simulink model "BLDCMODELTOTALNEURON"  (R2020a)
settings: Solver=ode45  StartTime=0.0  StopTime=2  RelTol=1e-3  EnableMultiTasking=on
InitFcn:
  | clc;
StopFcn:
  | clc;
undefined symbols (not defined in the file): sigbuilder_block, Ts
libraries: neural x55, fl_lib x14, nesl_utility x14, simulink x7, spsIGBTDiodeLib x6, spsVoltageMeasurementLib x3, powerlib_extras x1, spsControlledVoltageSourceLib x1, spsGroundLib x1, spsThreePhaseVIMeasurementLib x1, spspowerguiLib x1
(part 1 of 3)
Description:
  | This simulink model simulates the speed control of permanent magnet
  | brush less DC motor. Complete dynamic model of brush-less DC motor
  | was developed and simulated. Conventional PI controller was employed
  | for speed loop.
  | 
  | Syed Abdul Rahman Kashif
  | EED, UET, Lahore
settings Model: Creator=AbdulRahman  LastModifiedBy=HP
settings SolverCC: ZeroCrossAlgorithm=Adaptive
settings DataIOCC: LimitDataPoints=on  SaveFormat=Array  ReturnWorkspaceOutputs=off
settings OptimizationCC: ExpressionDepthLimit=2147483647  LifeSpan=inf
settings DebuggingCC: UnderspecifiedInitializationDetection=Classic  MergeDetectMultiDrivingBlocksExec=none  SolverPrmCheckMsg=warning  StateNameClashWarn=warning  SFUnexpectedBacktrackingDiag=warning  SFNoUnconditionalDefaultTransitionDiag=warning  ArithmeticOperatorsInVariantConditions=warning
settings HardwareCC: ProdBitPerPointer=32  ProdBitPerSizeT=32  ProdBitPerPtrDiffT=32  ProdLargestAtomicFloat=None  ProdIntDivRoundTo=Undefined  ProdEndianess=Unspecified  ProdWordSize=32  ProdHWDeviceType=32-bit Generic
settings ModelReferenceCC: PropagateSignalLabelsOutOfModel=off
settings SFSimCC: SimUseLocalCustomCode=off  CustomCodeUndefinedFunction=UseInterfaceOnly
settings RTWCC: RTWUseLocalCustomCode=off
settings CodeAppCC: StateflowObjectComments=on
settings GRTTargetCC: TargetLangStandard=C89/C90 (ANSI)
settings ConfigComp: CovMetricSettings=dw  CovSaveCumulativeToWorkspaceVar=on  CovSaveSingleToWorkspaceVar=on  CovExternalEMLEnable=off
settings SimscapeCC: SimscapeNormalizeSystem=off

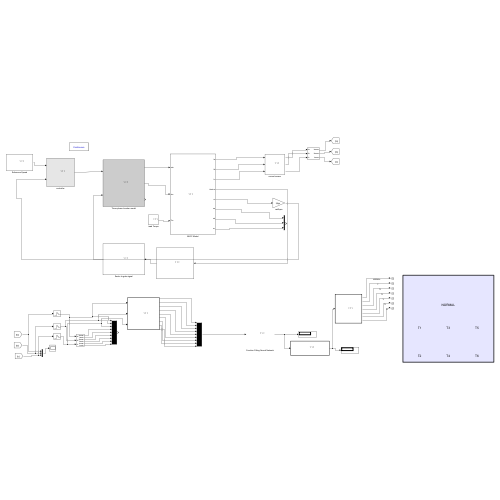
[thumbnail: Simulink's stored preview of the top-level diagram]
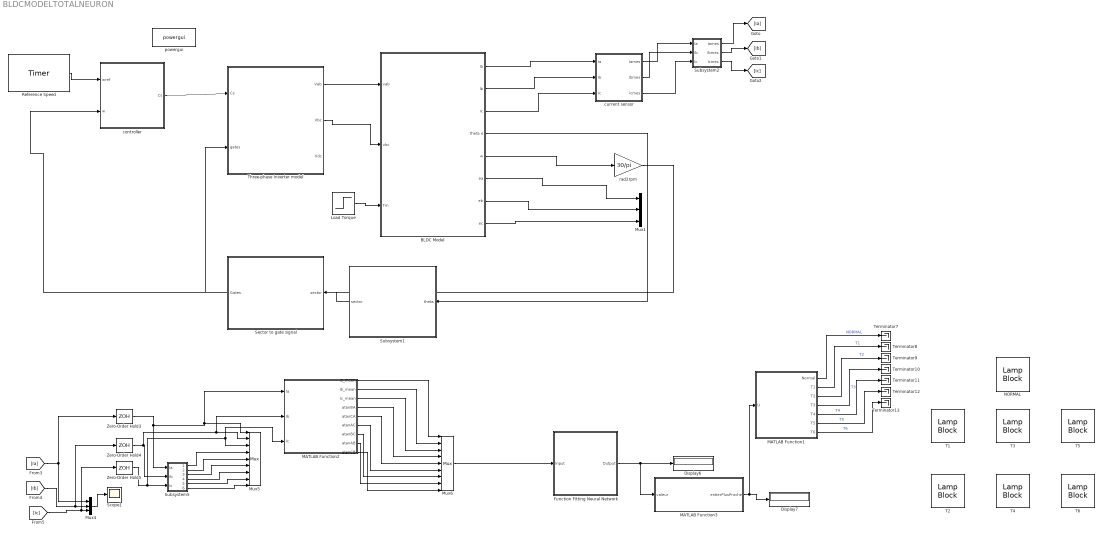
== system BLDCMODELTOTALNEURON ==
  BLDC Model : Subsystem
      mask Display: image(imread('C:\Users\HP\Desktop\2EEIN\PFATOTALYEAR\brush.png'))
  Display6 : Display
  Display7 : Display
  Function Fitting Neural Network : Subsystem
      mask help: Function Fitting Neural Network
      mask Display: image(imread('C:\Users\HP\Desktop\pythonpfa\neuron.png'))
  Load Torque : Step  Time=0.2  After=2  SampleTime=0
      mask Display: image(imread('C:\Users\HP\Desktop\2EEIN\PFATOTALYEAR\tor.png'))
  MATLAB Function1 : MATLAB Function  TreatAsAtomicUnit=on
  MATLAB Function2 : MATLAB Function  TreatAsAtomicUnit=on
  MATLAB Function3 : MATLAB Function  TreatAsAtomicUnit=on
  Mux1 : Mux  Inputs=3
  Mux4 : Mux  Inputs=3
  Mux5 : Mux  Inputs=9
  Mux6 : Mux  Inputs=9
  NORMAL : LampBlock
  Reference Speed : powerlib_extras/Control  Blocks/Timer  t=[0]  e=[1500]  mask(Timer){}
      settings: SourceProductBaseCode=PS
      mask Display:
      | % This is a new mask on top of the base mask.
      | % Use "View base mask" link below to see the base mask.
      | image(imread('C:\Users\HP\Desktop\2EEIN\PFATOTALYEAR\acc.png'))
  Scope1 : Scope
  Sector to gate signal : Subsystem
      mask Display: image(imread('C:\Users\HP\Desktop\2EEIN\PFATOTALYEAR\decoder.png'))
  Subsystem1 : Subsystem
      mask Display: image(imread('C:\Users\HP\Desktop\2EEIN\PFATOTALYEAR\sensor.png'))
  Subsystem2 : Subsystem
  Subsystem5 : Subsystem
  T{1..6} (6 alike) : LampBlock
  Terminator{7..13} (7 alike) : Terminator
  Three-phase Inverter model : Subsystem
      mask Display: image(imread('C:\Users\HP\Desktop\2EEIN\PFATOTALYEAR\threephase.png'))
  Zero-Order Hold3 : ZeroOrderHold  SampleTime=-1
  Zero-Order Hold4 : ZeroOrderHold  SampleTime=-1
  Zero-Order Hold5 : ZeroOrderHold  SampleTime=-1
  controller : Subsystem
      mask Display: image(imread('C:\Users\HP\Desktop\2EEIN\PFATOTALYEAR\pidcont.png'))
  current sensor : Subsystem
      mask Display: image(imread('C:\Users\HP\Desktop\2EEIN\PFATOTALYEAR\current.png'))
  powergui : spspowerguiLib/powergui  Priority=2  SimulationMode=Continuous  SampleTime=Ts  frequency=60  Iterations=50  frequencyindice=0  Pbase=100e6  ErrMax=1e-4  UnitsV=kV  UnitsW=MW  buscounter=0  FunctionMessages=off  echomessages=off  EnableUseOfTLC=off  CurrentSourceSwitches=off  DisableSnubberDevices=off  DisableRonSwitches=off  DisableVfSwitches=off  DisplayEquations=off  AutomaticDiscreteSolvers=off  SolverType=Tustin  Interpol=off  ExternalGateDelay=off  methode=off  Ts=0  x0status=blocks  SPID=off  SwTol=0  HookPort=off  NonlinearTolerance=1e-4  nMaxIteration=100  ContinueOnMaxIteration=off  RestoreLinks=warning  ResistiveCurrentMeasurement=off  Frange=[0:2:500]  Ylog=off  Xlog=on  ShowGrid=off  save=off  variable=ZData  structure=0  ZoomFFT=on  StartTime=0.0  cycles=1  DisplayStyle=1  fundamental=60  FreqAxis=off  MaxFrequency=1000  frequencyindicesteady=1  RmsSteady=1  display=off
  rad2rpm : Gain  Gain=30/pi
  wires:
  Subsystem1/1(sector) -> Sector to gate signal/1(sector)
  rad2rpm/1 -> controller/2(w)
  Reference Speed/1 -> controller/1(wref)
  Load Torque/1 -> BLDC Model/3(Tm)
  BLDC Model/5(w) -> rad2rpm/1
  BLDC Model/4(theta e) -> Subsystem1/1(theta)
  BLDC Model/6(ea) -> Mux1/1
  BLDC Model/7(eb) -> Mux1/2
  BLDC Model/8(ec) -> Mux1/3
  Sector to gate signal/1(Gates) -> Three-phase Inverter model/2(gates)
  controller/1(Cs) -> Three-phase Inverter model/1(Cs)
  Three-phase Inverter model/2(Vbc) -> BLDC Model/2(vbc)
  Three-phase Inverter model/1(Vab) -> BLDC Model/1(vab)
  BLDC Model/1(Ia) -> current sensor/1(Ia)
  BLDC Model/2(Ib) -> current sensor/2(Ib)
  BLDC Model/3(Ic) -> current sensor/3(Ic)
  current sensor/2(Ibmes) -> Subsystem2/2(Ib)
  Subsystem2/3(Icmes) -> [Ic]
  Subsystem2/1(Iames) -> [Ia]
  Subsystem2/2(Ibmes) -> [Ib]
  current sensor/1(Iames) -> Subsystem2/1(Ia)
  current sensor/3(Icmes) -> Subsystem2/3(Ic)
  Function Fitting Neural Network/1(Output) -> MATLAB Function3/1(valeur), Display6/1
  MATLAB Function2/2(Ib_mean) -> Mux6/2
  Zero-Order Hold3/1 -> MATLAB Function2/1(Ia), Mux5/1, Subsystem5/1(Ia)
  Zero-Order Hold4/1 -> MATLAB Function2/2(Ib), Mux5/2, Subsystem5/2(Ib)
  MATLAB Function2/3(Ic_mean) -> Mux6/3
  Subsystem5/3(Ibmax) -> Mux5/6
  Subsystem5/6(Icmin) -> Mux5/9
  [Ia] -> Zero-Order Hold3/1, Mux4/1
  [Ib] -> Zero-Order Hold4/1, Mux4/2
  Mux4/1 -> Scope1/1
  Mux6/1 -> Function Fitting Neural Network/1(Input)
  MATLAB Function2/6(atanAC) -> Mux6/6
  MATLAB Function2/5(atanCA) -> Mux6/5
  MATLAB Function2/4(atanBA) -> Mux6/4
  Zero-Order Hold5/1 -> MATLAB Function2/3(Ic), Mux5/3, Subsystem5/3(Ic)
  MATLAB Function2/9(atanCB) -> Mux6/9
  [Ic] -> Zero-Order Hold5/1, Mux4/3
  Subsystem5/4(Ibmin) -> Mux5/7
  Subsystem5/5(icmax) -> Mux5/8
  Subsystem5/1(Iamax) -> Mux5/4
  MATLAB Function2/7(atanBC) -> Mux6/7
  MATLAB Function2/8(atanAB) -> Mux6/8
  Subsystem5/2(Iamin) -> Mux5/5
  MATLAB Function2/1(Ia_mean) -> Mux6/1
  MATLAB Function3/1(entierPlusProche) -> MATLAB Function1/1(U), Display7/1
  MATLAB Function1/6(T5) -> Terminator12/1  "T5"
  MATLAB Function1/4(T3) -> Terminator10/1  "T3"
  MATLAB Function1/2(T1) -> Terminator8/1  "T1"
  MATLAB Function1/3(T2) -> Terminator9/1  "T2"
  MATLAB Function1/1(Normal) -> Terminator7/1  "NORMAL"
  MATLAB Function1/7(T6) -> Terminator13/1  "T6"
  MATLAB Function1/5(T4) -> Terminator11/1  "T4"

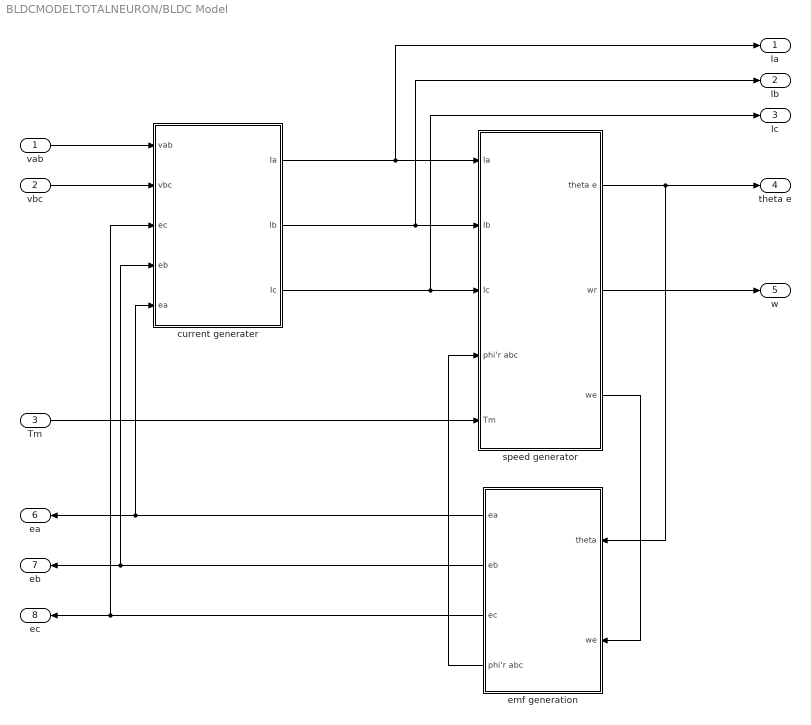
== system BLDCMODELTOTALNEURON/BLDC Model ==
  vab : Inport
  vbc : Inport  Port=2
  Tm : Inport  Port=3
  current generater : Subsystem
  emf generation : Subsystem
  speed generator : Subsystem
  Ia : Outport
  Ib : Outport  Port=2
  Ic : Outport  Port=3
  theta e : Outport  Port=4
  w : Outport  Port=5
  ea : Outport  Port=6
  eb : Outport  Port=7
  ec : Outport  Port=8
  wires:
  vbc/1 -> current generater/2(vbc)
  current generater/1(Ia) -> Ia/1, speed generator/1(Ia)
  current generater/2(Ib) -> Ib/1, speed generator/2(Ib)
  current generater/3(Ic) -> speed generator/3(Ic), Ic/1
  speed generator/1(theta e) -> emf generation/1(theta), theta e/1
  Tm/1 -> speed generator/5(Tm)
  speed generator/2(wr) -> w/1
  emf generation/1(ea) -> ea/1, current generater/5(ea)
  emf generation/2(eb) -> eb/1, current generater/4(eb)
  emf generation/3(ec) -> ec/1, current generater/3(ec)
  emf generation/4(phi'r abc) -> speed generator/4(phi'r abc)
  speed generator/3(we) -> emf generation/2(we)
  vab/1 -> current generater/1(vab)

== system BLDCMODELTOTALNEURON/Function Fitting Neural Network ==
  Input : Inport  PortDimensions=9
      mask Display: e = 0.06;c1 = [120 230 180]/255;c2 = ([120 230 180]+0)/(256+128);c3 = ([120 230 180]+128)/(256+128);patch([0 1 1 0],[0 0 1 1],c1);patch([0 1 1 1-e 1-e 0+e],[0 0 1 1-e 0+e 0+e],c2);patch([0 0 1 1-e 0+e 0+e],[0 1 1 1-e 1-e 0+e],c3);plot([0 1 1 0 0],[0 0 1 1 0]);
  Layer 1 : Subsystem
      mask Display: e = 0.06;c1 = [120 150 230]/255;c2 = ([120 150 230]+0)/383;c3 = ([120 150 230]+128)/383;patch([0 1 1 0],[0 0 1 1],c1);patch([0 1 1 1-e 1-e 0+e],[0 0 1 1-e 0+e 0+e],c2);patch([0 0 1 1-e 0+e 0+e],[0 1 1 1-e 1-e 0+e],c3);plot([0 1 1 0 0],[0 0 1 1 0]);
  Layer 2 : Subsystem
      mask Display: e = 0.06;c1 = [120 150 230]/255;c2 = ([120 150 230]+0)/383;c3 = ([120 150 230]+128)/383;patch([0 1 1 0],[0 0 1 1],c1);patch([0 1 1 1-e 1-e 0+e],[0 0 1 1-e 0+e 0+e],c2);patch([0 0 1 1-e 0+e 0+e],[0 1 1 1-e 1-e 0+e],c3);plot([0 1 1 0 0],[0 0 1 1 0]);
  Process Input 1 : Subsystem
      mask Display: e = 0.06;c1 = [120 150 230]/255;c2 = ([120 150 230]+0)/383;c3 = ([120 150 230]+128)/383;patch([0 1 1 0],[0 0 1 1],c1);patch([0 1 1 1-e 1-e 0+e],[0 0 1 1-e 0+e 0+e],c2);patch([0 0 1 1-e 0+e 0+e],[0 1 1 1-e 1-e 0+e],c3);plot([0 1 1 0 0],[0 0 1 1 0]);
  Process Output 1 : Subsystem
      mask Display: e = 0.06;c1 = [120 150 230]/255;c2 = ([120 150 230]+0)/383;c3 = ([120 150 230]+128)/383;patch([0 1 1 0],[0 0 1 1],c1);patch([0 1 1 1-e 1-e 0+e],[0 0 1 1-e 0+e 0+e],c2);patch([0 0 1 1-e 0+e 0+e],[0 1 1 1-e 1-e 0+e],c3);plot([0 1 1 0 0],[0 0 1 1 0]);
  Output : Outport  InitialOutput=0
      mask Display: e = 0.06;c1 = [120 230 180]/255;c2 = ([120 230 180]+0)/(256+128);c3 = ([120 230 180]+128)/(256+128);patch([0 1 1 0],[0 0 1 1],c1);patch([0 1 1 1-e 1-e 0+e],[0 0 1 1-e 0+e 0+e],c2);patch([0 0 1 1-e 0+e 0+e],[0 1 1 1-e 1-e 0+e],c3);plot([0 1 1 0 0],[0 0 1 1 0]);
  wires:
  Input/1 -> Process Input 1/1(x)
  Process Output 1/1(y) -> Output/1
  Process Input 1/1(p) -> Layer 1/1("p{1}")
  Layer 1/1("a{1}") -> [feedback1]
  [feedback1] -> Layer 2/1("a{1} ")
  Layer 2/1("a{2}") -> Process Output 1/1(a)

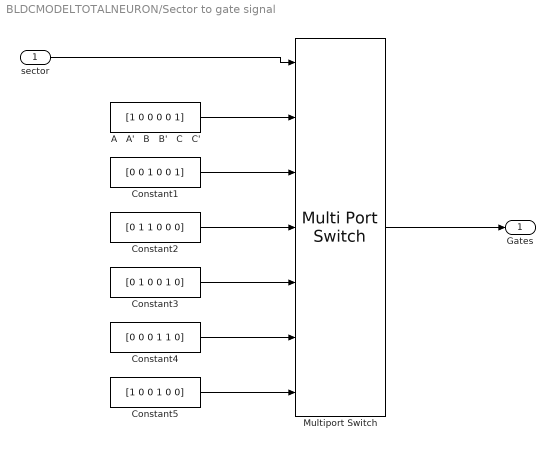
== system BLDCMODELTOTALNEURON/Sector to gate signal ==
  sector : Inport
  A   A'   B   B'   C   C' : Constant  Value=[1 0 0 0 0 1]  VectorParams1D=off
  Constant1 : Constant  Value=[0 0 1 0 0 1]  VectorParams1D=off
  Constant2 : Constant  Value=[0 1 1 0 0 0]  VectorParams1D=off
  Constant3 : Constant  Value=[0 1 0 0 1 0]  VectorParams1D=off
  Constant4 : Constant  Value=[0 0 0 1 1 0]  VectorParams1D=off
  Constant5 : Constant  Value=[1 0 0 1 0 0]  VectorParams1D=off
  Multiport Switch : MultiPortSwitch  Inputs=6
  Gates : Outport
  wires:
  Multiport Switch/1 -> Gates/1
  A   A'   B   B'   C   C'/1 -> Multiport Switch/2
  Constant1/1 -> Multiport Switch/3
  Constant2/1 -> Multiport Switch/4
  Constant3/1 -> Multiport Switch/5
  Constant4/1 -> Multiport Switch/6
  Constant5/1 -> Multiport Switch/7
  sector/1 -> Multiport Switch/1

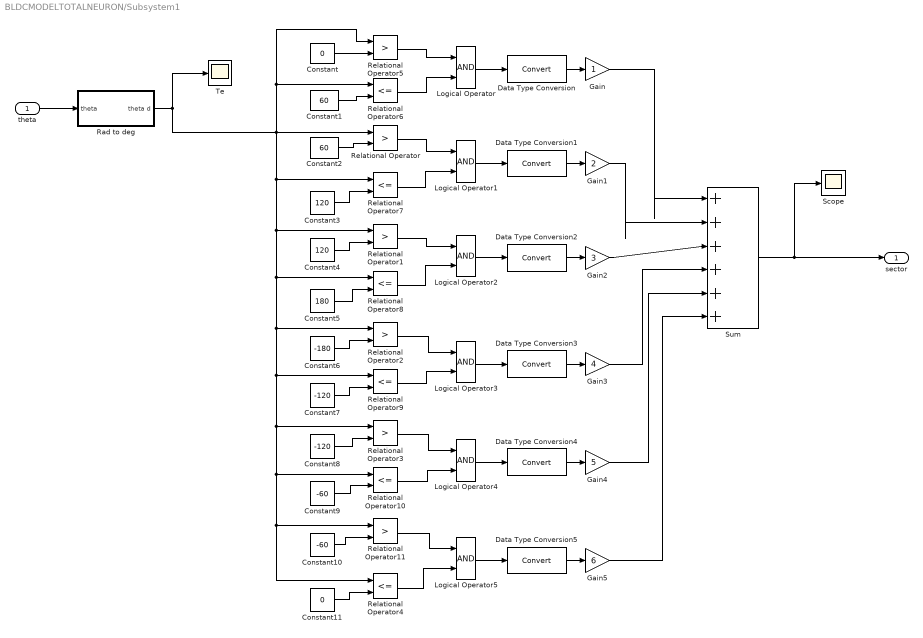
== system BLDCMODELTOTALNEURON/Subsystem1 ==
  theta : Inport
  Constant : Constant  Value=0
  Constant1 : Constant  Value=60
  Constant10 : Constant  Value=-60
  Constant11 : Constant  Value=0
  Constant2 : Constant  Value=60
  Constant3 : Constant  Value=120
  Constant4 : Constant  Value=120
  Constant5 : Constant  Value=180
  Constant6 : Constant  Value=-180
  Constant7 : Constant  Value=-120
  Constant8 : Constant  Value=-120
  Constant9 : Constant  Value=-60
  Data Type Conversion{,1..5} (6 alike) : DataTypeConversion
  Gain : Gain
  Gain1 : Gain  Gain=2
  Gain2 : Gain  Gain=3
  Gain3 : Gain  Gain=4
  Gain4 : Gain  Gain=5
  Gain5 : Gain  Gain=6
  Logical Operator{,1..5} (6 alike) : Logic  AllPortsSameDT=off  OutDataTypeStr=boolean
  Rad to deg : Subsystem
  Relational Operator{,1..3,5,11} (6 alike) : RelationalOperator  Operator=>  OutDataTypeStr=boolean  ZeroCross=off  RndMeth=Nearest
  Relational Operator{4,6..10} (6 alike) : RelationalOperator  Operator=<=  OutDataTypeStr=boolean  ZeroCross=off  RndMeth=Nearest
  Scope : Scope
  Sum : Sum  Inputs=|++++++
  Te : Scope
  sector : Outport
  wires:
  Sum/1 -> sector/1, Scope/1
  theta/1 -> Rad to deg/1(theta)
  Constant/1 -> Relational Operator5/2
  Constant1/1 -> Relational Operator6/2
  Constant2/1 -> Relational Operator/2
  Constant3/1 -> Relational Operator7/2
  Rad to deg/1(theta d) -> Relational Operator5/1, Relational Operator6/1, Relational Operator4/1, Relational Operator11/1, Relational Operator10/1, Relational Operator3/1, Relational Operator9/1, Relational Operator2/1, Relational Operator8/1, Relational Operator1/1, Relational Operator7/1, Relational Operator/1, Te/1
  Constant5/1 -> Relational Operator8/2
  Constant6/1 -> Relational Operator2/2
  Constant7/1 -> Relational Operator9/2
  Constant8/1 -> Relational Operator3/2
  Constant9/1 -> Relational Operator10/2
  Constant10/1 -> Relational Operator11/2
  Constant11/1 -> Relational Operator4/2
  Constant4/1 -> Relational Operator1/2
  Relational Operator11/1 -> Logical Operator5/1
  Relational Operator4/1 -> Logical Operator5/2
  Relational Operator3/1 -> Logical Operator4/1
  Relational Operator10/1 -> Logical Operator4/2
  Relational Operator2/1 -> Logical Operator3/1
  Relational Operator9/1 -> Logical Operator3/2
  Relational Operator5/1 -> Logical Operator/1
  Relational Operator6/1 -> Logical Operator/2
  Relational Operator/1 -> Logical Operator1/1
  Relational Operator7/1 -> Logical Operator1/2
  Relational Operator1/1 -> Logical Operator2/1
  Relational Operator8/1 -> Logical Operator2/2
  Gain4/1 -> Sum/5
  Gain3/1 -> Sum/4
  Gain5/1 -> Sum/6
  Gain2/1 -> Sum/3
  Gain1/1 -> Sum/2
  Gain/1 -> Sum/1
  Logical Operator/1 -> Data Type Conversion/1
  Data Type Conversion/1 -> Gain/1
  Data Type Conversion1/1 -> Gain1/1
  Logical Operator1/1 -> Data Type Conversion1/1
  Data Type Conversion2/1 -> Gain2/1
  Logical Operator2/1 -> Data Type Conversion2/1
  Data Type Conversion3/1 -> Gain3/1
  Logical Operator3/1 -> Data Type Conversion3/1
  Data Type Conversion4/1 -> Gain4/1
  Logical Operator4/1 -> Data Type Conversion4/1
  Data Type Conversion5/1 -> Gain5/1
  Logical Operator5/1 -> Data Type Conversion5/1

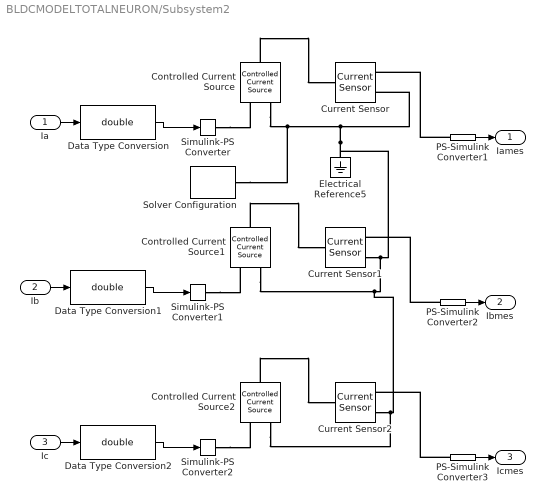
== system BLDCMODELTOTALNEURON/Subsystem2 ==
  Ia : Inport
  Ib : Inport  Port=2
  Ic : Inport  Port=3
  Controlled Current Source : fl_lib/Electrical/Electrical Sources/Controlled Current Source
  Controlled Current Source1 : fl_lib/Electrical/Electrical Sources/Controlled Current Source
  Controlled Current Source2 : fl_lib/Electrical/Electrical Sources/Controlled Current Source
  Current Sensor : fl_lib/Electrical/Electrical Sensors/Current Sensor
  Current Sensor1 : fl_lib/Electrical/Electrical Sensors/Current Sensor
  Current Sensor2 : fl_lib/Electrical/Electrical Sensors/Current Sensor
  Data Type Conversion : DataTypeConversion  OutDataTypeStr=double
  Data Type Conversion1 : DataTypeConversion  OutDataTypeStr=double
  Data Type Conversion2 : DataTypeConversion  OutDataTypeStr=double
  Electrical Reference5 : fl_lib/Electrical/Electrical Elements/Electrical Reference
  PS-Simulink Converter1 : nesl_utility/PS-Simulink Converter  PhysicalDomain=network_engine_domain  SubClassName=ps_output  LeftPortType=input  RightPortType=output  PseudoPeriodic=off  Frequencies=[]  Unit=inherit  AffineConversion=off
      settings: SourceProductBaseCode=PW,SS
  PS-Simulink Converter2 : nesl_utility/PS-Simulink Converter  PhysicalDomain=network_engine_domain  SubClassName=ps_output  LeftPortType=input  RightPortType=output  PseudoPeriodic=off  Frequencies=[]  Unit=inherit  AffineConversion=off
      settings: SourceProductBaseCode=PW,SS
  PS-Simulink Converter3 : nesl_utility/PS-Simulink Converter  PhysicalDomain=network_engine_domain  SubClassName=ps_output  LeftPortType=input  RightPortType=output  PseudoPeriodic=off  Frequencies=[]  Unit=inherit  AffineConversion=off
      settings: SourceProductBaseCode=PW,SS
  Simulink-PS Converter : nesl_utility/Simulink-PS Converter  PhysicalDomain=network_engine_domain  SubClassName=ps_input  LeftPortType=input  RightPortType=output  PseudoPeriodic=off  Frequencies=[]  NoiseDistribution=none  NoiseParameters=[]  Unit=1  AffineConversion=off  FilteringAndDerivatives=provide  SimscapeFilterOrder=1  InputFilterTimeConstant=0.001  UdotUserProvided=0
      settings: SourceProductBaseCode=PW,SS
  Simulink-PS Converter1 : nesl_utility/Simulink-PS Converter  PhysicalDomain=network_engine_domain  SubClassName=ps_input  LeftPortType=input  RightPortType=output  PseudoPeriodic=off  Frequencies=[]  NoiseDistribution=none  NoiseParameters=[]  Unit=1  AffineConversion=off  FilteringAndDerivatives=provide  SimscapeFilterOrder=1  InputFilterTimeConstant=0.001  UdotUserProvided=0
      settings: SourceProductBaseCode=PW,SS
  Simulink-PS Converter2 : nesl_utility/Simulink-PS Converter  PhysicalDomain=network_engine_domain  SubClassName=ps_input  LeftPortType=input  RightPortType=output  PseudoPeriodic=off  Frequencies=[]  NoiseDistribution=none  NoiseParameters=[]  Unit=1  AffineConversion=off  FilteringAndDerivatives=provide  SimscapeFilterOrder=1  InputFilterTimeConstant=0.001  UdotUserProvided=0
      settings: SourceProductBaseCode=PW,SS
  Solver Configuration : nesl_utility/Solver Configuration  PhysicalDomain=network_engine_domain  SubClassName=solver  LeftPortType=input  RightPortType=generic  Tones=[]  Harmonics=[]  SimulateNoise=off  Profile=off  UseLocalSampling=off  EnableSwitchedLinearOptims=on  FrequencyDomain=off  UseCCode=off  RelTol=0.001  AbsTol=1e-06  MinStep=1e-09  ToWorkspace=off  RevertToSquareIcSolve=off  NumHomotopyIterations=100  PhasorMode=off  PhasorModeNumHarmonics=1  DoDC=off  ResidualTolerance=1e-09  UseLocalSolver=off  LocalSolverChoice=NE_BACKWARD_EULER_ADVANCER  LocalSolverSampleTime=0.001  DoFixedCost=off  MaxNonlinIter=3  MaxModeIter=2  ComputeImpulses=off  ImpulseIterations=2  LinearAlgebra=auto  EquationFormulation=NE_TIME_EF  DelaysMemoryBudget=1024  AutomaticFiltering=on  FilteringTimeConstant=0.001  PartitionStorageMethod=AS_NEEDED  PartitionMemoryBudget=1024  PartitionMethod=ROBUST
      settings: SourceProductBaseCode=PW,SS
  Iames : Outport
  Ibmes : Outport  Port=2
  Icmes : Outport  Port=3
  wires:
  PS-Simulink Converter1/1 -> Iames/1
  Data Type Conversion/1 -> Simulink-PS Converter/1
  Ia/1 -> Data Type Conversion/1
  PS-Simulink Converter2/1 -> Ibmes/1
  Ib/1 -> Data Type Conversion1/1
  Data Type Conversion1/1 -> Simulink-PS Converter1/1
  PS-Simulink Converter3/1 -> Icmes/1
  Ic/1 -> Data Type Conversion2/1
  Data Type Conversion2/1 -> Simulink-PS Converter2/1
  connections:
  Controlled Current Source/RConn2 -- Solver Configuration/RConn1 -- Controlled Current Source2/RConn2 -- Current Sensor2/RConn2 -- Controlled Current Source1/RConn2 -- Current Sensor1/RConn2 -- Electrical Reference5/LConn1 -- Current Sensor/RConn2
  Controlled Current Source/LConn1 -- Current Sensor/LConn1
  Simulink-PS Converter/RConn1 -- Controlled Current Source/RConn1
  PS-Simulink Converter1/LConn1 -- Current Sensor/RConn1
  Controlled Current Source1/LConn1 -- Current Sensor1/LConn1
  Simulink-PS Converter1/RConn1 -- Controlled Current Source1/RConn1
  PS-Simulink Converter2/LConn1 -- Current Sensor1/RConn1
  Controlled Current Source2/LConn1 -- Current Sensor2/LConn1
  Simulink-PS Converter2/RConn1 -- Controlled Current Source2/RConn1
  PS-Simulink Converter3/LConn1 -- Current Sensor2/RConn1

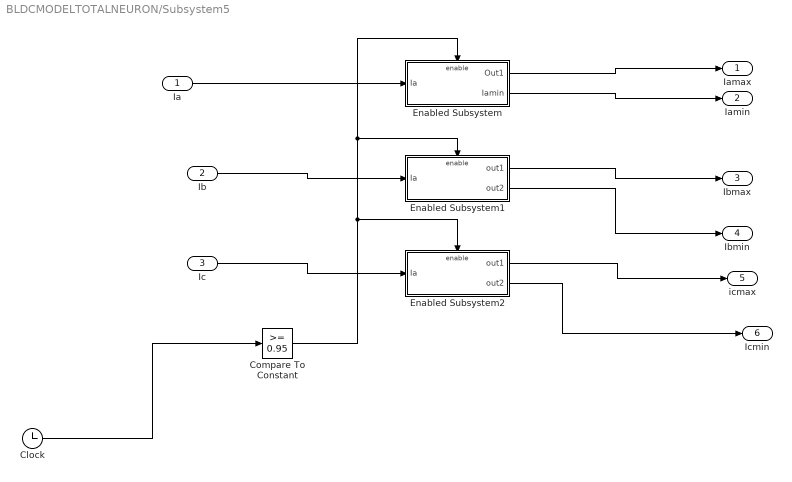
== system BLDCMODELTOTALNEURON/Subsystem5 ==
  Ia : Inport
  Ib : Inport  Port=2
  Ic : Inport  Port=3
  Clock : Clock
  Compare To Constant : simulink/Logic and Bit Operations/Compare To Constant  relop=>=  const=0.95  OutDataTypeStr=boolean
  Enabled Subsystem : Subsystem  TreatAsAtomicUnit=on
  Enabled Subsystem1 : Subsystem  TreatAsAtomicUnit=on
  Enabled Subsystem2 : Subsystem  TreatAsAtomicUnit=on
  Iamax : Outport
  Iamin : Outport  Port=2
  Ibmax : Outport  Port=3
  Ibmin : Outport  Port=4
  icmax : Outport  Port=5
  Icmin : Outport  Port=6
  wires:
  Clock/1 -> Compare To Constant/1
  Ia/1 -> Enabled Subsystem/1(Ia)
  Ic/1 -> Enabled Subsystem2/1(Ia)
  Ib/1 -> Enabled Subsystem1/1(Ia)
  Compare To Constant/1 -> Enabled Subsystem2/Enable, Enabled Subsystem1/Enable, Enabled Subsystem/Enable
  Enabled Subsystem/1(Out1) -> Iamax/1
  Enabled Subsystem/2(Iamin) -> Iamin/1
  Enabled Subsystem1/1(out1) -> Ibmax/1
  Enabled Subsystem1/2(out2) -> Ibmin/1
  Enabled Subsystem2/1(out1) -> icmax/1
  Enabled Subsystem2/2(out2) -> Icmin/1

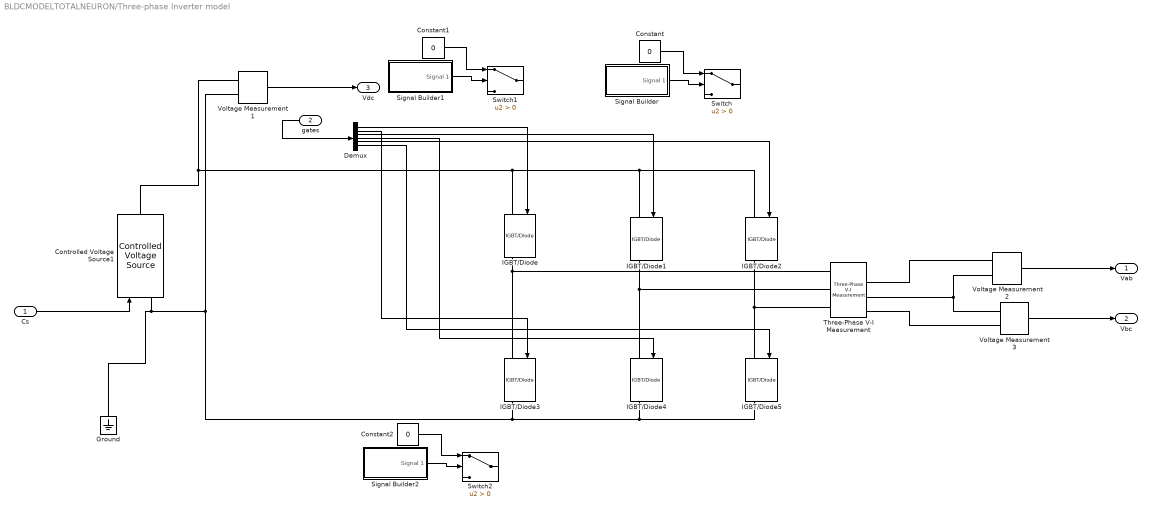
== system BLDCMODELTOTALNEURON/Three-phase Inverter model ==
  Cs : Inport
  gates : Inport  Port=2
  Constant : Constant  Value=0
  Constant1 : Constant  Value=0
  Constant2 : Constant  Value=0
  Controlled Voltage Source1 : spsControlledVoltageSourceLib/Controlled Voltage Source  Initialize=on  Source_Type=DC  Amplitude=500  Phase=0  Frequency=0  Measurements=None
  Demux : Demux  Outputs=6
  Ground : spsGroundLib/Ground  LConnTagsString=a
  IGBT/Diode{,1..5} (6 alike) : spsIGBTDiodeLib/IGBT//Diode  Ron=1e-3  Rs=5000  Cs=1e-6  Measurements=on
  Signal Builder : Subsystem  Tag=STV Subsys  LoadFcn=sigbuilder_block('load');  StartFcn=sigbuilder_block('start');  StopFcn=sigbuilder_block('stop');  ClipboardFcn=sigbuilder_block('clipboard');  mask(Sigbuilder block){tuvar=[0:10]}
      mask help: Simulink:masks:SigbuilderBlock_MD
      mask init:
      | if ~strcmp(get_param(bdroot(gcbh),'SimulationStatus'),'stopped') tuvar = sigbuilder_block('maskInit'); end
      settings: CopyFcn=sigbuilder_block('copy');  DeleteFcn=sigbuilder_block('delete');  ModelCloseFcn=sigbuilder_block('modelClose');  PreSaveFcn=sigbuilder_block('preSave');  PauseFcn=sigbuilder_block('pause');  ContinueFcn=sigbuilder_block('continue');  NameChangeFcn=sigbuilder_block('namechange');  OpenFcn=sigbuilder_block('open',[437.6 199.2 550.4 400 ]);  CloseFcn=sigbuilder_block('close');
      mask Display: plot(0, 0, 100, 100,[2, 2, 32, 32, 2], [68, 8, 8, 68, 68],[32, 2], [38, 38], [32, 19, 2],[53, 60, 44], [32, 17, 17, 2],[16, 16, 31, 31]);txt = getActiveGroup(gcbh);text(2, 100, txt,'verticalAlignment', 'top');
  Signal Builder1 : Subsystem  Tag=STV Subsys  LoadFcn=sigbuilder_block('load');  StartFcn=sigbuilder_block('start');  StopFcn=sigbuilder_block('stop');  ClipboardFcn=sigbuilder_block('clipboard');  mask(Sigbuilder block){tuvar=[0:10]}
      mask help: Simulink:masks:SigbuilderBlock_MD
      mask init:
      | if ~strcmp(get_param(bdroot(gcbh),'SimulationStatus'),'stopped') tuvar = sigbuilder_block('maskInit'); end
      settings: CopyFcn=sigbuilder_block('copy');  DeleteFcn=sigbuilder_block('delete');  ModelCloseFcn=sigbuilder_block('modelClose');  PreSaveFcn=sigbuilder_block('preSave');  PauseFcn=sigbuilder_block('pause');  ContinueFcn=sigbuilder_block('continue');  NameChangeFcn=sigbuilder_block('namechange');  OpenFcn=sigbuilder_block('open',[437.6 199.2 550.4 400 ]);  CloseFcn=sigbuilder_block('close');
      mask Display: plot(0, 0, 100, 100,[2, 2, 32, 32, 2], [68, 8, 8, 68, 68],[32, 2], [38, 38], [32, 19, 2],[53, 60, 44], [32, 17, 17, 2],[16, 16, 31, 31]);txt = getActiveGroup(gcbh);text(2, 100, txt,'verticalAlignment', 'top');
  Signal Builder2 : Subsystem  Tag=STV Subsys  LoadFcn=sigbuilder_block('load');  StartFcn=sigbuilder_block('start');  StopFcn=sigbuilder_block('stop');  ClipboardFcn=sigbuilder_block('clipboard');  mask(Sigbuilder block){tuvar=[0:10]}
      mask help: Simulink:masks:SigbuilderBlock_MD
      mask init:
      | if ~strcmp(get_param(bdroot(gcbh),'SimulationStatus'),'stopped') tuvar = sigbuilder_block('maskInit'); end
      settings: CopyFcn=sigbuilder_block('copy');  DeleteFcn=sigbuilder_block('delete');  ModelCloseFcn=sigbuilder_block('modelClose');  PreSaveFcn=sigbuilder_block('preSave');  PauseFcn=sigbuilder_block('pause');  ContinueFcn=sigbuilder_block('continue');  NameChangeFcn=sigbuilder_block('namechange');  OpenFcn=sigbuilder_block('open',[437.6 199.2 550.4 400 ]);  CloseFcn=sigbuilder_block('close');
      mask Display: plot(0, 0, 100, 100,[2, 2, 32, 32, 2], [68, 8, 8, 68, 68],[32, 2], [38, 38], [32, 19, 2],[53, 60, 44], [32, 17, 17, 2],[16, 16, 31, 31]);txt = getActiveGroup(gcbh);text(2, 100, txt,'verticalAlignment', 'top');
  Switch : Switch  Criteria=u2 > Threshold
  Switch1 : Switch  Criteria=u2 > Threshold
  Switch2 : Switch  Criteria=u2 > Threshold
  Three-Phase V-I Measurement : spsThreePhaseVIMeasurementLib/Three-Phase V-I Measurement  VoltageMeasurement=phase-to-ground  SetLabelV=off  LabelV=Vabc  Vpu=off  VpuLL=off  CurrentMeasurement=no  SetLabelI=off  LabelI=Iabc  Ipu=off  Pbase=100e6  Vbase=500e3  OutputType=Complex  PhasorSimulation=off  PSBequivalent=0
  Voltage Measurement1 : spsVoltageMeasurementLib/Voltage Measurement  PhasorSimulation=off  OutputType=Complex  PSBequivalent=0
  Voltage Measurement2 : spsVoltageMeasurementLib/Voltage Measurement  PhasorSimulation=off  OutputType=Complex  PSBequivalent=0
      link override source: GotoTag=tp96803dc0_013b_4907_89cd_69d70f818148
  Voltage Measurement3 : spsVoltageMeasurementLib/Voltage Measurement  PhasorSimulation=off  OutputType=Complex  PSBequivalent=0
  Vab : Outport
  Vbc : Outport  Port=2
  Vdc : Outport  Port=3
  wires:
  Cs/1 -> Controlled Voltage Source1/1
  Voltage Measurement1/1 -> Vdc/1
  gates/1 -> Demux/1
  Voltage Measurement2/1 -> Vab/1
  Voltage Measurement3/1 -> Vbc/1
  Signal Builder/1(Signal 1) -> Switch/2
  Constant/1 -> Switch/1
  Constant1/1 -> Switch1/1
  Signal Builder1/1(Signal 1) -> Switch1/2
  Signal Builder2/1(Signal 1) -> Switch2/2
  Constant2/1 -> Switch2/1
  Demux/5 -> IGBT/Diode2/1
  Demux/4 -> IGBT/Diode4/1
  Demux/6 -> IGBT/Diode5/1
  Demux/3 -> IGBT/Diode1/1
  Demux/1 -> IGBT/Diode/1
  Demux/2 -> IGBT/Diode3/1
  connections:
  Controlled Voltage Source1/RConn1 -- IGBT/Diode/LConn1 -- IGBT/Diode1/LConn1 -- IGBT/Diode2/LConn1 -- Voltage Measurement1/LConn1
  Controlled Voltage Source1/LConn1 -- IGBT/Diode5/RConn1 -- IGBT/Diode4/RConn1 -- IGBT/Diode3/RConn1 -- Voltage Measurement1/LConn2 -- Ground/LConn1
  Voltage Measurement3/LConn1 -- Three-Phase V-I Measurement/RConn2 -- Voltage Measurement2/LConn2
  IGBT/Diode/RConn1 -- Three-Phase V-I Measurement/LConn1 -- IGBT/Diode3/LConn1
  IGBT/Diode2/RConn1 -- Three-Phase V-I Measurement/LConn3 -- IGBT/Diode5/LConn1
  IGBT/Diode1/RConn1 -- Three-Phase V-I Measurement/LConn2 -- IGBT/Diode4/LConn1
  Three-Phase V-I Measurement/RConn1 -- Voltage Measurement2/LConn1
  Three-Phase V-I Measurement/RConn3 -- Voltage Measurement3/LConn2

== system BLDCMODELTOTALNEURON/controller ==
  wref : Inport
  w : Inport  Port=2
  Add : Sum
  Gain : Gain  Gain=0.1
  Gain1 : Gain  Gain=50
  Integrator : Integrator
  Sum : Sum  Inputs=|+-
  Cs : Outport
  wires:
  wref/1 -> Sum/1
  w/1 -> Sum/2
  Add/1 -> Cs/1
  Sum/1 -> Gain1/1, Gain/1
  Gain1/1 -> Integrator/1
  Gain/1 -> Add/1
  Integrator/1 -> Add/2

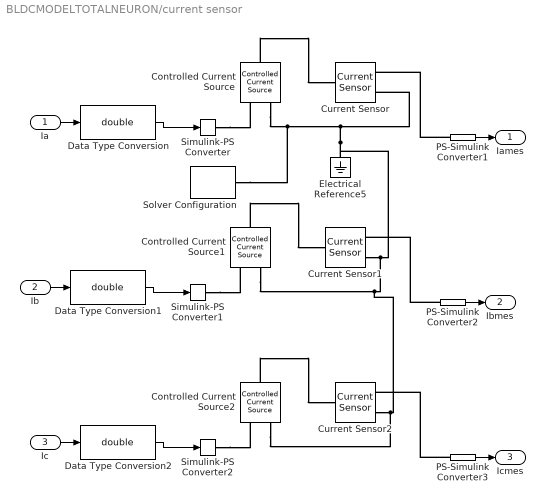
== system BLDCMODELTOTALNEURON/current sensor ==
  Ia : Inport
  Ib : Inport  Port=2
  Ic : Inport  Port=3
  Controlled Current Source : fl_lib/Electrical/Electrical Sources/Controlled Current Source
  Controlled Current Source1 : fl_lib/Electrical/Electrical Sources/Controlled Current Source
  Controlled Current Source2 : fl_lib/Electrical/Electrical Sources/Controlled Current Source
  Current Sensor : fl_lib/Electrical/Electrical Sensors/Current Sensor
  Current Sensor1 : fl_lib/Electrical/Electrical Sensors/Current Sensor
  Current Sensor2 : fl_lib/Electrical/Electrical Sensors/Current Sensor
  Data Type Conversion : DataTypeConversion  OutDataTypeStr=double
  Data Type Conversion1 : DataTypeConversion  OutDataTypeStr=double
  Data Type Conversion2 : DataTypeConversion  OutDataTypeStr=double
  Electrical Reference5 : fl_lib/Electrical/Electrical Elements/Electrical Reference
  PS-Simulink Converter1 : nesl_utility/PS-Simulink Converter  PhysicalDomain=network_engine_domain  SubClassName=ps_output  LeftPortType=input  RightPortType=output  PseudoPeriodic=off  Frequencies=[]  Unit=inherit  AffineConversion=off
      settings: SourceProductBaseCode=PW,SS
  PS-Simulink Converter2 : nesl_utility/PS-Simulink Converter  PhysicalDomain=network_engine_domain  SubClassName=ps_output  LeftPortType=input  RightPortType=output  PseudoPeriodic=off  Frequencies=[]  Unit=inherit  AffineConversion=off
      settings: SourceProductBaseCode=PW,SS
  PS-Simulink Converter3 : nesl_utility/PS-Simulink Converter  PhysicalDomain=network_engine_domain  SubClassName=ps_output  LeftPortType=input  RightPortType=output  PseudoPeriodic=off  Frequencies=[]  Unit=inherit  AffineConversion=off
      settings: SourceProductBaseCode=PW,SS
  Simulink-PS Converter : nesl_utility/Simulink-PS Converter  PhysicalDomain=network_engine_domain  SubClassName=ps_input  LeftPortType=input  RightPortType=output  PseudoPeriodic=off  Frequencies=[]  NoiseDistribution=none  NoiseParameters=[]  Unit=1  AffineConversion=off  FilteringAndDerivatives=provide  SimscapeFilterOrder=1  InputFilterTimeConstant=0.001  UdotUserProvided=0
      settings: SourceProductBaseCode=PW,SS
  Simulink-PS Converter1 : nesl_utility/Simulink-PS Converter  PhysicalDomain=network_engine_domain  SubClassName=ps_input  LeftPortType=input  RightPortType=output  PseudoPeriodic=off  Frequencies=[]  NoiseDistribution=none  NoiseParameters=[]  Unit=1  AffineConversion=off  FilteringAndDerivatives=provide  SimscapeFilterOrder=1  InputFilterTimeConstant=0.001  UdotUserProvided=0
      settings: SourceProductBaseCode=PW,SS
  Simulink-PS Converter2 : nesl_utility/Simulink-PS Converter  PhysicalDomain=network_engine_domain  SubClassName=ps_input  LeftPortType=input  RightPortType=output  PseudoPeriodic=off  Frequencies=[]  NoiseDistribution=none  NoiseParameters=[]  Unit=1  AffineConversion=off  FilteringAndDerivatives=provide  SimscapeFilterOrder=1  InputFilterTimeConstant=0.001  UdotUserProvided=0
      settings: SourceProductBaseCode=PW,SS
  Solver Configuration : nesl_utility/Solver Configuration  PhysicalDomain=network_engine_domain  SubClassName=solver  LeftPortType=input  RightPortType=generic  Tones=[]  Harmonics=[]  SimulateNoise=off  Profile=off  UseLocalSampling=off  EnableSwitchedLinearOptims=on  FrequencyDomain=off  UseCCode=off  RelTol=0.001  AbsTol=1e-06  MinStep=1e-09  ToWorkspace=off  RevertToSquareIcSolve=off  NumHomotopyIterations=100  PhasorMode=off  PhasorModeNumHarmonics=1  DoDC=off  ResidualTolerance=1e-09  UseLocalSolver=off  LocalSolverChoice=NE_BACKWARD_EULER_ADVANCER  LocalSolverSampleTime=0.001  DoFixedCost=off  MaxNonlinIter=3  MaxModeIter=2  ComputeImpulses=off  ImpulseIterations=2  LinearAlgebra=auto  EquationFormulation=NE_TIME_EF  DelaysMemoryBudget=1024  AutomaticFiltering=on  FilteringTimeConstant=0.001  PartitionStorageMethod=AS_NEEDED  PartitionMemoryBudget=1024  PartitionMethod=ROBUST
      settings: SourceProductBaseCode=PW,SS
  Iames : Outport
  Ibmes : Outport  Port=2
  Icmes : Outport  Port=3
  wires:
  PS-Simulink Converter1/1 -> Iames/1
  Data Type Conversion/1 -> Simulink-PS Converter/1
  Ia/1 -> Data Type Conversion/1
  PS-Simulink Converter2/1 -> Ibmes/1
  Ib/1 -> Data Type Conversion1/1
  Data Type Conversion1/1 -> Simulink-PS Converter1/1
  PS-Simulink Converter3/1 -> Icmes/1
  Ic/1 -> Data Type Conversion2/1
  Data Type Conversion2/1 -> Simulink-PS Converter2/1
  connections:
  Controlled Current Source/RConn2 -- Solver Configuration/RConn1 -- Controlled Current Source2/RConn2 -- Current Sensor2/RConn2 -- Controlled Current Source1/RConn2 -- Current Sensor1/RConn2 -- Electrical Reference5/LConn1 -- Current Sensor/RConn2
  Controlled Current Source/LConn1 -- Current Sensor/LConn1
  Simulink-PS Converter/RConn1 -- Controlled Current Source/RConn1
  PS-Simulink Converter1/LConn1 -- Current Sensor/RConn1
  Controlled Current Source1/LConn1 -- Current Sensor1/LConn1
  Simulink-PS Converter1/RConn1 -- Controlled Current Source1/RConn1
  PS-Simulink Converter2/LConn1 -- Current Sensor1/RConn1
  Controlled Current Source2/LConn1 -- Current Sensor2/LConn1
  Simulink-PS Converter2/RConn1 -- Controlled Current Source2/RConn1
  PS-Simulink Converter3/LConn1 -- Current Sensor2/RConn1

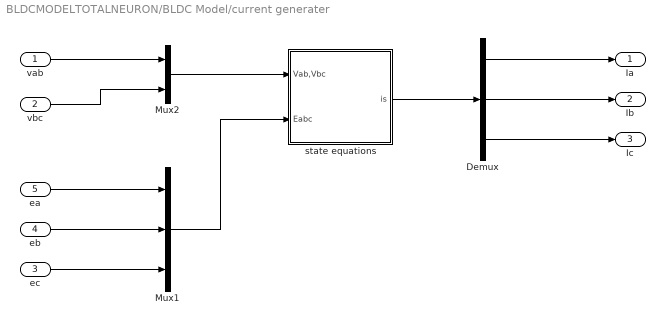
== system BLDCMODELTOTALNEURON/BLDC Model/current generater ==
  vab : Inport
  vbc : Inport  Port=2
  ec : Inport  Port=3
  eb : Inport  Port=4
  ea : Inport  Port=5
  Demux : Demux  Outputs=3
  Mux1 : Mux  Inputs=3
  Mux2 : Mux  Inputs=2
  state equations : Subsystem
  Ia : Outport
  Ib : Outport  Port=2
  Ic : Outport  Port=3
  wires:
  state equations/1(is) -> Demux/1
  ea/1 -> Mux1/1
  eb/1 -> Mux1/2
  ec/1 -> Mux1/3
  Mux1/1 -> state equations/2(Eabc)
  Demux/1 -> Ia/1
  Demux/2 -> Ib/1
  Demux/3 -> Ic/1
  vab/1 -> Mux2/1
  vbc/1 -> Mux2/2
  Mux2/1 -> state equations/1(Vab,Vbc)

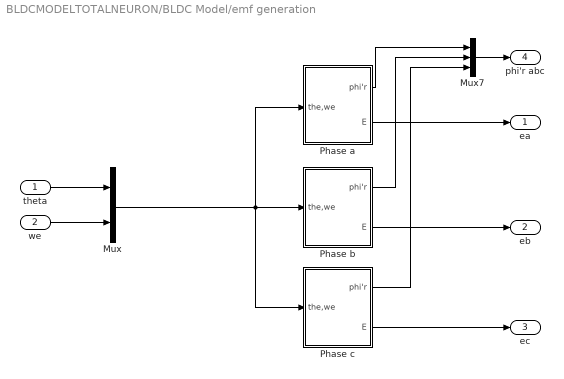
== system BLDCMODELTOTALNEURON/BLDC Model/emf generation ==
  theta : Inport
  we : Inport  Port=2
  Mux : Mux  Inputs=2
  Mux7 : Mux  Inputs=3
  Phase a : Subsystem
  Phase b : Subsystem
  Phase c : Subsystem
  ea : Outport
  eb : Outport  Port=2
  ec : Outport  Port=3
  phi'r abc : Outport  Port=4
  wires:
  Mux7/1 -> phi'r abc/1
  Phase c/1(phi'r) -> Mux7/3
  Phase b/1(phi'r) -> Mux7/2
  Phase a/1(phi'r) -> Mux7/1
  Mux/1 -> Phase a/1(the,we), Phase b/1(the,we), Phase c/1(the,we)
  Phase a/2(E) -> ea/1
  Phase b/2(E) -> eb/1
  Phase c/2(E) -> ec/1
  theta/1 -> Mux/1
  we/1 -> Mux/2

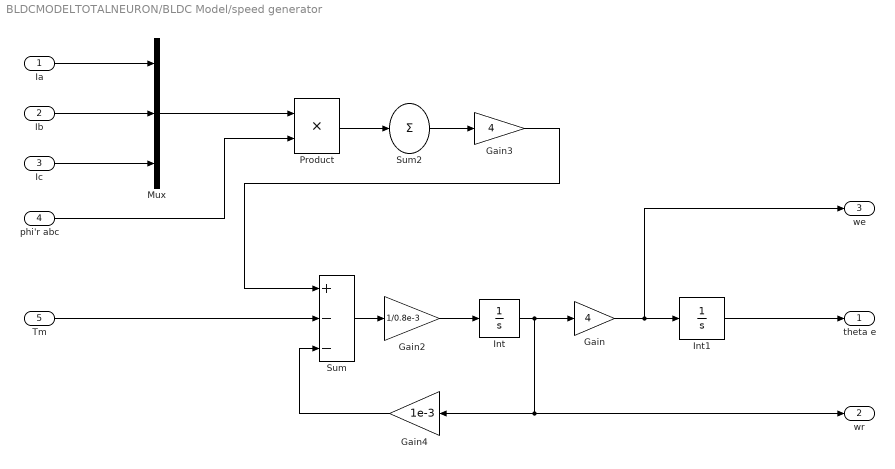
== system BLDCMODELTOTALNEURON/BLDC Model/speed generator ==
  Ia : Inport
  Ib : Inport  Port=2
  Ic : Inport  Port=3
  phi'r abc : Inport  Port=4
  Tm : Inport  Port=5
  Gain : Gain  Gain=4  SaturateOnIntegerOverflow=on  OutDataTypeStr=Inherit: Same as input  ParamDataTypeStr=Inherit: Same as input
  Gain2 : Gain  Gain=1/0.8e-3  SaturateOnIntegerOverflow=on  OutDataTypeStr=Inherit: Same as input  ParamDataTypeStr=Inherit: Same as input
  Gain3 : Gain  Gain=4  SaturateOnIntegerOverflow=on  OutDataTypeStr=Inherit: Same as input  ParamDataTypeStr=Inherit: Same as input
  Gain4 : Gain  Gain=1e-3  SaturateOnIntegerOverflow=on  OutDataTypeStr=Inherit: Same as input  ParamDataTypeStr=Inherit: Same as input
  Int : Integrator
  Int1 : Integrator
  Mux : Mux  Inputs=3
  Product : Product  SaturateOnIntegerOverflow=on  OutDataTypeStr=Inherit: Same as first input
  Sum : Sum  Inputs=+--  InputSameDT=on  SaturateOnIntegerOverflow=on  OutDataTypeStr=Inherit: Same as first input
  Sum2 : Sum  Inputs=+  SaturateOnIntegerOverflow=on
  theta e : Outport
  wr : Outport  Port=2
  we : Outport  Port=3
  wires:
  Ia/1 -> Mux/1
  Ib/1 -> Mux/2
  Ic/1 -> Mux/3
  Gain3/1 -> Sum/1
  Sum2/1 -> Gain3/1
  Product/1 -> Sum2/1
  Mux/1 -> Product/1
  phi'r abc/1 -> Product/2
  Int1/1 -> theta e/1
  Gain/1 -> Int1/1, we/1
  Int/1 -> Gain/1, Gain4/1, wr/1
  Gain2/1 -> Int/1
  Sum/1 -> Gain2/1
  Gain4/1 -> Sum/3
  Tm/1 -> Sum/2

== system BLDCMODELTOTALNEURON/Function Fitting Neural Network/Layer 1 ==
  "p{1}" : Inport  PortDimensions=9
      mask Display: e = 0.06;c1 = [120 230 180]/255;c2 = ([120 230 180]+0)/(256+128);c3 = ([120 230 180]+128)/(256+128);patch([0 1 1 0],[0 0 1 1],c1);patch([0 1 1 1-e 1-e 0+e],[0 0 1 1-e 0+e 0+e],c2);patch([0 0 1 1-e 0+e 0+e],[0 1 1 1-e 1-e 0+e],c3);plot([0 1 1 0 0],[0 0 1 1 0]);
  Delays 1 : Subsystem
      mask Display: e = 0.06;c1 = [120 150 230]/255;c2 = ([120 150 230]+0)/383;c3 = ([120 150 230]+128)/383;patch([0 1 1 0],[0 0 1 1],c1);patch([0 1 1 1-e 1-e 0+e],[0 0 1 1-e 0+e 0+e],c2);patch([0 0 1 1-e 0+e 0+e],[0 1 1 1-e 1-e 0+e],c3);plot([0 1 1 0 0],[0 0 1 1 0]);disp('0');
  "IW{1,1}" : Subsystem
      mask Display: e = 0.06;c1 = [120 150 230]/255;c2 = ([120 150 230]+0)/383;c3 = ([120 150 230]+128)/383;patch([0 1 1 0],[0 0 1 1],c1);patch([0 1 1 1-e 1-e 0+e],[0 0 1 1-e 0+e 0+e],c2);patch([0 0 1 1-e 0+e 0+e],[0 1 1 1-e 1-e 0+e],c3);plot([0 1 1 0 0],[0 0 1 1 0]);disp('W');
  "b{1}" : Constant  Value=[-3.793354691290600211317496359697543084621429443359375;7.87157172203525501430476651876233518123626708984375;-5.09166043220916808564879829646088182926177978515625;-8.27735572553837783971175667829811573028564453125;-3.134195527817769999501251731999218463897705078125;2.72283868210453494640432836604304611682891845703125;-0.49164903368906731628840134362690150737762451171875;-0.72680014931897030106000556770595721900463104248046875;7.946944915556390043320789118297398090362548828125;0.0105771402768698487284471099201255128718912601470947265625;-0.9425140298282357331771663666586391627788543701171875;-3.53249118083051172334307921119034290313720703125;4.2018102270859056801555198035202920436859130859375;-3.395199615100485512897421358502469956874847412109375;3.189750692353578553905890657915733754634857177734375;6.578098082270276591998481308110058307647705078125;-1.4643413194806900179401054629124701023101806640625;0.2209443257778218872022790719711338169872760772705078125;5.09616671964097012192951297038234770298004150390625;-2.001511982652020460449193706153891980648040771484375;-3.0784631810844249599767863401211798191070556640625;6.64676629181839384585828156559728085994720458984375;2.243346427372161056013055713265202939510345458984375;3.051765393377924073803342253086157143115997314453125;5.747354674415504405260435305535793304443359375;2.078416268542204736746725757257081568241119384765625;0.07483551802358294480210787469331989996135234832763671875;-1.7481042404246991406324696072260849177837371826171875;4.37553532750710072463107280782423913478851318359375;58.3652395314730796371804899536073207855224609375;-1.651140911751782791583309517591260373592376708984375;-3.922873612414921495883390889503061771392822265625;-5.5852061397170462697658877004869282245635986328125;6.40396580460138498125388650805689394474029541015625;15.811360813120682422550089540891349315643310546875;-2.917952645051529625419561853050254285335540771484375;7.44666694703578091463214150280691683292388916015625;-2.09683134069916565778157746535725891590118408203125;14.7459705121445718845052397227846086025238037109375;-1.8380437127692494936326284005190245807170867919921875;0.347299719766303083279268548722029663622379302978515625;9.0903749870358669937786544323898851871490478515625;-6.538410851843675430927760316990315914154052734375;-5.91480555286983200602435317705385386943817138671875;7.81734808472940567725117944064550101757049560546875;-1.9340820261787017297905322266160510480403900146484375;-2.948161473530839682410942259593866765499114990234375;4.96908758191990163055606899433769285678863525390625;-19.5005341571519039689519559033215045928955078125;8.9165807646776489292506084893830120563507080078125]
      mask Display: e = 0.06;c1 = [120 150 230]/255;c2 = ([120 150 230]+0)/383;c3 = ([120 150 230]+128)/383;patch([0 1 1 0],[0 0 1 1],c1);patch([0 1 1 1-e 1-e 0+e],[0 0 1 1-e 0+e 0+e],c2);patch([0 0 1 1-e 0+e 0+e],[0 1 1 1-e 1-e 0+e],c3);plot([0 1 1 0 0],[0 0 1 1 0]);disp('b');
  netsum : Sum  Inputs=2  InputSameDT=on  SaturateOnIntegerOverflow=on  OutDataTypeStr=Inherit: Same as first input
      mask Display: e = 0.06;c1 = [120 150 230]/255;c2 = ([120 150 230]+0)/383;c3 = ([120 150 230]+128)/383;patch([0 1 1 0],[0 0 1 1],c1);patch([0 1 1 1-e 1-e 0+e],[0 0 1 1-e 0+e 0+e],c2);patch([0 0 1 1-e 0+e 0+e],[0 1 1 1-e 1-e 0+e],c3);plot([0 1 1 0 0],[0 0 1 1 0]);disp('+');
  tansig : neural/Transfer Functions/tansig
  "a{1}" : Outport  InitialOutput=[0;0;0;0;0;0;0;0;0;0;0;0;0;0;0;0;0;0;0;0;0;0;0;0;0;0;0;0;0;0;0;0;0;0;0;0;0;0;0;0;0;0;0;0;0;0;0;0;0;0]
      mask Display: e = 0.06;c1 = [120 230 180]/255;c2 = ([120 230 180]+0)/(256+128);c3 = ([120 230 180]+128)/(256+128);patch([0 1 1 0],[0 0 1 1],c1);patch([0 1 1 1-e 1-e 0+e],[0 0 1 1-e 0+e 0+e],c2);patch([0 0 1 1-e 0+e 0+e],[0 1 1 1-e 1-e 0+e],c3);plot([0 1 1 0 0],[0 0 1 1 0]);
  wires:
  "p{1}"/1 -> Delays 1/1("p{1}")
  Delays 1/1("pd{1,1}") -> "IW{1,1}"/1("pd{1,1}")
  "IW{1,1}"/1("iz{1,1}") -> netsum/1
  "b{1}"/1 -> netsum/2
  netsum/1 -> tansig/1
  tansig/1 -> "a{1}"/1

== system BLDCMODELTOTALNEURON/Function Fitting Neural Network/Layer 2 ==
  "a{1} " : Inport  PortDimensions=50
      mask Display: e = 0.06;c1 = [120 230 180]/255;c2 = ([120 230 180]+0)/(256+128);c3 = ([120 230 180]+128)/(256+128);patch([0 1 1 0],[0 0 1 1],c1);patch([0 1 1 1-e 1-e 0+e],[0 0 1 1-e 0+e 0+e],c2);patch([0 0 1 1-e 0+e 0+e],[0 1 1 1-e 1-e 0+e],c3);plot([0 1 1 0 0],[0 0 1 1 0]);
  Delays 1 : Subsystem
      mask Display: e = 0.06;c1 = [120 150 230]/255;c2 = ([120 150 230]+0)/383;c3 = ([120 150 230]+128)/383;patch([0 1 1 0],[0 0 1 1],c1);patch([0 1 1 1-e 1-e 0+e],[0 0 1 1-e 0+e 0+e],c2);patch([0 0 1 1-e 0+e 0+e],[0 1 1 1-e 1-e 0+e],c3);plot([0 1 1 0 0],[0 0 1 1 0]);disp('0');
  "LW{2,1}" : Subsystem
      mask Display: e = 0.06;c1 = [120 150 230]/255;c2 = ([120 150 230]+0)/383;c3 = ([120 150 230]+128)/383;patch([0 1 1 0],[0 0 1 1],c1);patch([0 1 1 1-e 1-e 0+e],[0 0 1 1-e 0+e 0+e],c2);patch([0 0 1 1-e 0+e 0+e],[0 1 1 1-e 1-e 0+e],c3);plot([0 1 1 0 0],[0 0 1 1 0]);disp('W');
  "b{2}" : Constant  Value=0.5840169153360281750764215757953934371471405029296875
      mask Display: e = 0.06;c1 = [120 150 230]/255;c2 = ([120 150 230]+0)/383;c3 = ([120 150 230]+128)/383;patch([0 1 1 0],[0 0 1 1],c1);patch([0 1 1 1-e 1-e 0+e],[0 0 1 1-e 0+e 0+e],c2);patch([0 0 1 1-e 0+e 0+e],[0 1 1 1-e 1-e 0+e],c3);plot([0 1 1 0 0],[0 0 1 1 0]);disp('b');
  netsum : Sum  Inputs=2  InputSameDT=on  SaturateOnIntegerOverflow=on  OutDataTypeStr=Inherit: Same as first input
      mask Display: e = 0.06;c1 = [120 150 230]/255;c2 = ([120 150 230]+0)/383;c3 = ([120 150 230]+128)/383;patch([0 1 1 0],[0 0 1 1],c1);patch([0 1 1 1-e 1-e 0+e],[0 0 1 1-e 0+e 0+e],c2);patch([0 0 1 1-e 0+e 0+e],[0 1 1 1-e 1-e 0+e],c3);plot([0 1 1 0 0],[0 0 1 1 0]);disp('+');
  purelin : neural/Transfer Functions/purelin
  "a{2}" : Outport  InitialOutput=0
      mask Display: e = 0.06;c1 = [120 230 180]/255;c2 = ([120 230 180]+0)/(256+128);c3 = ([120 230 180]+128)/(256+128);patch([0 1 1 0],[0 0 1 1],c1);patch([0 1 1 1-e 1-e 0+e],[0 0 1 1-e 0+e 0+e],c2);patch([0 0 1 1-e 0+e 0+e],[0 1 1 1-e 1-e 0+e],c3);plot([0 1 1 0 0],[0 0 1 1 0]);
  wires:
  "a{1} "/1 -> Delays 1/1("p{2}")
  Delays 1/1("pd{2,1}") -> "LW{2,1}"/1("ad{2,1}")
  "LW{2,1}"/1("lz{2,1}") -> netsum/1
  "b{2}"/1 -> netsum/2
  netsum/1 -> purelin/1
  purelin/1 -> "a{2}"/1

== system BLDCMODELTOTALNEURON/Function Fitting Neural Network/Process Input 1 ==
  x : Inport  PortDimensions=9
      mask Display: e = 0.06;c1 = [120 230 180]/255;c2 = ([120 230 180]+0)/(256+128);c3 = ([120 230 180]+128)/(256+128);patch([0 1 1 0],[0 0 1 1],c1);patch([0 1 1 1-e 1-e 0+e],[0 0 1 1-e 0+e 0+e],c2);patch([0 0 1 1-e 0+e 0+e],[0 1 1 1-e 1-e 0+e],c3);plot([0 1 1 0 0],[0 0 1 1 0]);
  mapminmax : neural/Processing Functions/mapminmax  xmin=[-50375.4110226824996061623096466;-11335.9604090675893530715256929;-255127.589030852395808324217796;-141.718340448206390647101216018;-149.117896427192306418874068186;-153.607668226073712958168471232;-173.571367965800192223468911834;-128.573413897321586318867048249;-179.405538449769892395124770701]  xmax=[165466.47206434971303679049015;151357.762519892188720405101776;5995.59794915940710779977962375;160.012351181700211100178421475;157.68691743816191319638164714;158.612824655217707459087250754;165.447563321523205104313092306;174.737861994169605850402149372;173.890404524319507117979810573]  ymin=-1  ymax=1
  p : Outport  PortDimensions=9
      mask Display: e = 0.06;c1 = [120 230 180]/255;c2 = ([120 230 180]+0)/(256+128);c3 = ([120 230 180]+128)/(256+128);patch([0 1 1 0],[0 0 1 1],c1);patch([0 1 1 1-e 1-e 0+e],[0 0 1 1-e 0+e 0+e],c2);patch([0 0 1 1-e 0+e 0+e],[0 1 1 1-e 1-e 0+e],c3);plot([0 1 1 0 0],[0 0 1 1 0]);
  wires:
  x/1 -> mapminmax/1
  mapminmax/1 -> p/1

== system BLDCMODELTOTALNEURON/Function Fitting Neural Network/Process Output 1 ==
  a : Inport  PortDimensions=1
      mask Display: e = 0.06;c1 = [120 230 180]/255;c2 = ([120 230 180]+0)/(256+128);c3 = ([120 230 180]+128)/(256+128);patch([0 1 1 0],[0 0 1 1],c1);patch([0 1 1 1-e 1-e 0+e],[0 0 1 1-e 0+e 0+e],c2);patch([0 0 1 1-e 0+e 0+e],[0 1 1 1-e 1-e 0+e],c3);plot([0 1 1 0 0],[0 0 1 1 0]);
  mapminmax_reverse : neural/Processing Functions/mapminmax_reverse  xmin=1  xmax=190  ymin=-1  ymax=1
  y : Outport  PortDimensions=1
      mask Display: e = 0.06;c1 = [120 230 180]/255;c2 = ([120 230 180]+0)/(256+128);c3 = ([120 230 180]+128)/(256+128);patch([0 1 1 0],[0 0 1 1],c1);patch([0 1 1 1-e 1-e 0+e],[0 0 1 1-e 0+e 0+e],c2);patch([0 0 1 1-e 0+e 0+e],[0 1 1 1-e 1-e 0+e],c3);plot([0 1 1 0 0],[0 0 1 1 0]);
  wires:
  a/1 -> mapminmax_reverse/1
  mapminmax_reverse/1 -> y/1

== system BLDCMODELTOTALNEURON/Subsystem1/Rad to deg ==
  theta : Inport
  Te : Scope
  Te1 : Scope
  Trigonometric Function : Trigonometry
  Trigonometric Function1 : Trigonometry  Operator=cos
  Trigonometric Function2 : Trigonometry  Operator=atan2
  rad2deg : Gain  Gain=180/pi  SaturateOnIntegerOverflow=on  OutDataTypeStr=Inherit: Same as input  ParamDataTypeStr=Inherit: Same as input
  theta d : Outport
  wires:
  theta/1 -> Te1/1, Trigonometric Function/1, Trigonometric Function1/1
  Trigonometric Function/1 -> Trigonometric Function2/1
  Trigonometric Function1/1 -> Trigonometric Function2/2
  Trigonometric Function2/1 -> Te/1, rad2deg/1
  rad2deg/1 -> theta d/1

== system BLDCMODELTOTALNEURON/Subsystem5/Enabled Subsystem ==
  Ia : Inport
  Enable : EnablePort
  MinMax Running Resettable : simulink/Math Operations/MinMax Running Resettable  Function=max  vinit=0
  MinMax Running Resettable1 : simulink/Math Operations/MinMax Running Resettable  Function=min  vinit=0
  Out1 : Outport
  Iamin : Outport  Port=2
  wires:
  Ia/1 -> MinMax Running Resettable1/1, MinMax Running Resettable/1
  MinMax Running Resettable/1 -> Out1/1
  MinMax Running Resettable1/1 -> Iamin/1

== system BLDCMODELTOTALNEURON/Subsystem5/Enabled Subsystem1 ==
  Ia : Inport
  Enable : EnablePort
  MinMax Running Resettable : simulink/Math Operations/MinMax Running Resettable  Function=max  vinit=0
  MinMax Running Resettable1 : simulink/Math Operations/MinMax Running Resettable  Function=max  vinit=0
  out1 : Outport
  out2 : Outport  Port=2
  wires:
  Ia/1 -> MinMax Running Resettable1/1, MinMax Running Resettable/1
  MinMax Running Resettable/1 -> out1/1
  MinMax Running Resettable1/1 -> out2/1

== system BLDCMODELTOTALNEURON/Subsystem5/Enabled Subsystem2 ==
  Ia : Inport
  Enable : EnablePort
  MinMax Running Resettable : simulink/Math Operations/MinMax Running Resettable  Function=max  vinit=0
  MinMax Running Resettable1 : simulink/Math Operations/MinMax Running Resettable  Function=min  vinit=0
  out1 : Outport
  out2 : Outport  Port=2
  wires:
  Ia/1 -> MinMax Running Resettable1/1, MinMax Running Resettable/1
  MinMax Running Resettable/1 -> out1/1
  MinMax Running Resettable1/1 -> out2/1

== system BLDCMODELTOTALNEURON/Three-phase Inverter model/Signal Builder ==
  Demux : Demux  Tag=STV Demux  Outputs=1
      settings: DisplayOption=none
  FromWs : FromWorkspace  Tag=STV FromWs  VariableName=tuvar
      SigBuilderData=|
      | common.afterFinalStr = 'Extrapolate'
      | common.sampleTime = 0
      | dataSet.timeRange = [0 10]
      | dataSet.name = 'Group 1'
      | sbobj.Groups.Name = 'Group 1'
      | sbobj.Groups.Signals.Name = 'Signal 1'
      | sbobj.Groups.Signals.XData = [0 2 2 10]
      | sbobj.Groups.Signals.YData = [1 1 0 0]
  Signal 1 : Outport  Tag=STV Outport
  wires:
  Demux/1 -> Signal 1/1
  FromWs/1 -> Demux/1

== system BLDCMODELTOTALNEURON/Three-phase Inverter model/Signal Builder1 ==
  Demux : Demux  Tag=STV Demux  Outputs=1
      settings: DisplayOption=none
  FromWs : FromWorkspace  Tag=STV FromWs  VariableName=tuvar
      SigBuilderData=|
      | common.afterFinalStr = 'Extrapolate'
      | common.sampleTime = 0
      | dataSet.timeRange = [0 10]
      | dataSet.name = 'Group 1'
      | sbobj.Groups.Name = 'Group 1'
      | sbobj.Groups.Signals.Name = 'Signal 1'
      | sbobj.Groups.Signals.XData = [0 2 2 10]
      | sbobj.Groups.Signals.YData = [1 1 0 0]
  Signal 1 : Outport  Tag=STV Outport
  wires:
  Demux/1 -> Signal 1/1
  FromWs/1 -> Demux/1

== system BLDCMODELTOTALNEURON/Three-phase Inverter model/Signal Builder2 ==
  Demux : Demux  Tag=STV Demux  Outputs=1
      settings: DisplayOption=none
  FromWs : FromWorkspace  Tag=STV FromWs  VariableName=tuvar
      SigBuilderData=|
      | common.afterFinalStr = 'Extrapolate'
      | common.sampleTime = 0
      | dataSet.timeRange = [0 10]
      | dataSet.name = 'Group 1'
      | sbobj.Groups.Name = 'Group 1'
      | sbobj.Groups.Signals.Name = 'Signal 1'
      | sbobj.Groups.Signals.XData = [0 5.98 5.98 10]
      | sbobj.Groups.Signals.YData = [1.015 1 0 0]
  Signal 1 : Outport  Tag=STV Outport
  wires:
  Demux/1 -> Signal 1/1
  FromWs/1 -> Demux/1

== system BLDCMODELTOTALNEURON/BLDC Model/current generater/state equations ==
  Vab,Vbc : Inport
  Eabc : Inport  Port=2
  Mux5 : Mux  Inputs=3
  State Ib : Subsystem
  Sum1 : Sum  Inputs=--  SaturateOnIntegerOverflow=on
  state Ia : Subsystem
  is : Outport
  wires:
  Mux5/1 -> is/1
  Eabc/1 -> state Ia/2(Eabc), State Ib/2(Eabc)
  Sum1/1 -> Mux5/3
  State Ib/1(i) -> Sum1/2, Mux5/2
  state Ia/1(i) -> Sum1/1, Mux5/1
  Vab,Vbc/1 -> state Ia/1(Vab,Vbc), State Ib/1(Vab,Vbc)

== system BLDCMODELTOTALNEURON/BLDC Model/emf generation/Phase a ==
  note: Phi' r
  the,we : Inport
  Demux : Demux  Outputs=2
      settings: DisplayOption=none
  Gain4 : Gain  Gain=0.175  SaturateOnIntegerOverflow=on  OutDataTypeStr=Inherit: Same as input  ParamDataTypeStr=Inherit: Same as input
  Product1 : Product  SaturateOnIntegerOverflow=on  OutDataTypeStr=Inherit: Same as first input
  cos (u(1)) : Subsystem
  phi'r : Outport
  E : Outport  Port=2
  wires:
  Gain4/1 -> Product1/1, phi'r/1
  Product1/1 -> E/1
  the,we/1 -> Demux/1
  Demux/2 -> Product1/2
  Demux/1 -> cos (u(1))/1(In1)
  cos (u(1))/1(Out1) -> Gain4/1

== system BLDCMODELTOTALNEURON/BLDC Model/emf generation/Phase b ==
  note: Phi' r
  the,we : Inport
  Demux : Demux  Outputs=2
      settings: DisplayOption=none
  Gain4 : Gain  Gain=0.175  SaturateOnIntegerOverflow=on  OutDataTypeStr=Inherit: Same as input  ParamDataTypeStr=Inherit: Same as input
  Product1 : Product  SaturateOnIntegerOverflow=on  OutDataTypeStr=Inherit: Same as first input
  cos (u(1)) : Subsystem
  phi'r : Outport
  E : Outport  Port=2
  wires:
  cos (u(1))/1(Out1) -> Gain4/1
  Demux/1 -> cos (u(1))/1(In1)
  Demux/2 -> Product1/2
  the,we/1 -> Demux/1
  Product1/1 -> E/1
  Gain4/1 -> phi'r/1, Product1/1
